simulink model "Erdorbits"  (R2014b)
settings: Solver=ode45  StartTime=0.0  StopTime=86400  RelTol=1e-3
settings Model: Creator=hollowman  LastModifiedBy=sigurd

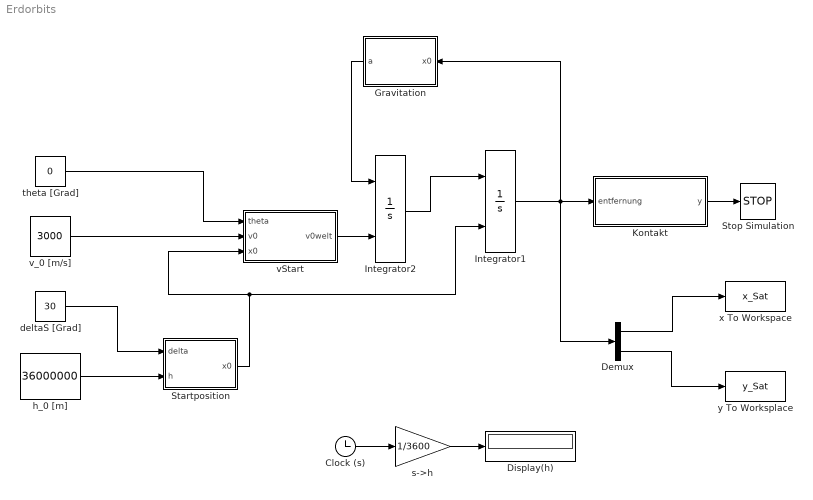
== system Erdorbits ==
  Clock (s) : Clock
  Demux : Demux  Outputs=2
  Display(h) : Display
  Gravitation : MATLAB Function  TreatAsAtomicUnit=on
  Integrator1 : Integrator  InitialConditionSource=external
  Integrator2 : Integrator  InitialConditionSource=external
  Kontakt : MATLAB Function  TreatAsAtomicUnit=on
  Startposition : MATLAB Function  TreatAsAtomicUnit=on
  Stop Simulation : Stop
  deltaS [Grad] : Constant  Value=30
  h_0 [m] : Constant  Value=36000000
  s->h : Gain  Gain=1/3600
  theta [Grad] : Constant  Value=0
  vStart : MATLAB Function  TreatAsAtomicUnit=on
  v_0 [m/s] : Constant  Value=3000
  x To Workspace : ToWorkspace  VariableName=x_Sat  SampleTime=-1
  y To Worksplace : ToWorkspace  VariableName=y_Sat  SampleTime=-1
  wires:
  Clock (s)/1 -> s->h/1
  s->h/1 -> Display(h)/1
  Demux/1 -> x To Workspace/1
  Demux/2 -> y To Worksplace/1
  Kontakt/1(y) -> Stop Simulation/1
  h_0 [m]/1 -> Startposition/2(h)
  deltaS [Grad]/1 -> Startposition/1(delta)
  Startposition/1(x0) -> vStart/3(x0), Integrator1/2
  theta [Grad]/1 -> vStart/1(theta)
  v_0 [m/s]/1 -> vStart/2(v0)
  Integrator1/1 -> Gravitation/1(x0), Demux/1, Kontakt/1(entfernung)
  vStart/1(v0welt) -> Integrator2/2
  Gravitation/1(a) -> Integrator2/1
  Integrator2/1 -> Integrator1/1

== matlab function Erdorbits/Startposition ==
  data: delta input; x0 output; h input
function x0 = fcn(delta, h)
er = 6378000; %Erdradius in Meter
bogen_delta = delta * pi / 180;
x  = cos(bogen_delta) * (er + h); 
y  = sin(bogen_delta) * (er + h);
%# Startposition als Spaltenvektor
x0 = [x ; y]

== matlab function Erdorbits/vStart ==
  data: theta input; v0 input; x0 input; v0welt output
function v0welt = fcn(theta, v0, x0)

bogen_theta = theta * pi / 180;

normE = x0 / norm(x0);              % Einheitsvektor in Normalrichtung
tanE = [normE(2) ; -normE(1)];      % Einheitsvektor in Tangentialrichtung (90 Grad gedreht)

t = cos(bogen_theta) * v0;          % Tangentialkomponente
n = sin(bogen_theta) * v0;          % Normalkomponente

v0welt = (t * tanE) + (n * normE);  % Geschwindigkeitsvektor

== matlab function Erdorbits/Gravitation ==
  data: x0 input; a output
function a = fcn(x0)

% Fs = m * a
% a = Fs / m
G = 66.7 * 10^(-12); % Gravitationskonstante
m_Erde = 5.9 * 10^24; % Masse der Erde

r_Erde = norm(x0); % Entfernung zur Erde

richtung = -x0 / r_Erde;
% Gravitationsbeschleunigung: a = m * G / r^2
a = richtung * (G * m_Erde /(r_Erde)^2)

== matlab function Erdorbits/Kontakt ==
  data: entfernung input; y output
function y = fcn(entfernung)
entfernung = norm(entfernung);

if(entfernung<=6378000)
    y = 1;
else
    y = 0;
end;
